simulink library "lib_FDM"  (R2019b)
settings: Solver=VariableStepAuto  StartTime=0.0  StopTime=10.0  RelTol=1e-3
values from neighbouring files (symbols this model uses):
  d = config.d_m    [computeTF.m]
undefined symbols (not defined in the file or in its folder): c_b_WGS, c_flat, c_grav, c_rot, c_rsma, Cd0, Cdcl, Cdcl2, Cl0, Cla, Cld, Cma, Cmd, Cmq, Cnb, Cnd, Cnr, Cra, Crd, Crp, Cy0, Cyb, Cyd, dmdt, Earth, HIL_Data, InitThrust, launchPos, me, mf, mp, Sref, tb, TF, theta0, WGS84
libraries: simulink_extras x14, $bdroot x7, simulink x5, lib_Fin_Deflections x3, aerolibasang x2, sharedtransform x1, aerolibtransform2 x1, aerolibbdyn x1, aerolibatmos2 x1, aerolibutil x1, aerolib6dof2 x1
(part 2 of 8)

== system lib_FDM/FDM/FDM_Linear/State_Integration ==
  FDM_States_Dot : Inport  OutDataTypeStr=Bus: FDM_States_Dot_Bus
  Simulation_Control : Inport  Port=2  OutDataTypeStr=Bus: Simulation_Ctrl_Bus
  States_Init : Inport  Port=3  OutDataTypeStr=Bus: States_Bus
  ATT_Integration : Subsystem
  Bus Creator : BusCreator  Inputs=4  OutDataTypeStr=Bus: FDM_States_Bus
  Bus Creator1 : BusCreator  Inputs=3  OutDataTypeStr=Bus: ATT_Euler_Bus
  Bus Creator2 : BusCreator  Inputs=3  OutDataTypeStr=Bus: Translation_States_Bus
  Bus Creator3 : BusCreator  Inputs=2  OutDataTypeStr=Bus: Airframe_States_Bus
  Bus Creator4 : BusCreator  Inputs=3  OutDataTypeStr=Bus: POS_WGS84_Bus
  Bus Creator5 : BusCreator  Inputs=3  OutDataTypeStr=Bus: POS_NED_Bus
  Bus Creator6 : BusCreator  Inputs=2  OutDataTypeStr=Bus: Position_States_Bus
  Bus Selector : BusSelector  OutputSignals=ATT_Euler_Dot.ATT_Dot_Phi_radDs,ATT_Euler_Dot.ATT_Dot_Theta_radDs,ATT_Euler_Dot.ATT_Dot_Psi_radDs
  Bus Selector1 : BusSelector  OutputSignals=Translation_States_Dot.ACC_x_B_mDs2,Translation_States_Dot.ACC_y_B_mDs2,Translation_States_Dot.ACC_z_B_mDs2
  Bus Selector2 : BusSelector  OutputSignals=Airframe_States_Dot.Motor_state_dot_percDs
  Bus Selector3 : BusSelector  OutputSignals=Position_States_Dot.POS_WGS84_Dot.POS_lambda_Dot_WGS84_radDs,Position_States_Dot.POS_WGS84_Dot.POS_mue_Dot_WGS84_radDs,Position_States_Dot.POS_WGS84_Dot.POS_h_Dot_WGS84_mDs
  Bus Selector4 : BusSelector  OutputSignals=Position_States_Dot.POS_NED_Dot.POS_x_Dot_NED_mDs,Position_States_Dot.POS_NED_Dot.POS_y_Dot_NED_mDs,Position_States_Dot.POS_NED_Dot.POS_z_Dot_NED_mDs
  Mass_Balance : Subsystem
  Motor_State_Integration : Subsystem
  POS_NED_Integrator : Subsystem
  POS_WGS84_Integrator : Subsystem
  Terminator1 : Terminator
  Terminator2 : Terminator
  Terminator3 : Terminator
  VEL_Integrator : Subsystem
  "FDM_States " : Outport  OutDataTypeStr=Bus: FDM_States_Bus  VectorParamsAs1DForOutWhenUnconnected=off
  wires:
  Mass_Balance/4(I_z_kgm2) -> Terminator3/1
  Mass_Balance/2(I_x_kgm2) -> Terminator1/1
  Mass_Balance/3(I_y_kgm2) -> Terminator2/1
  FDM_States_Dot/1 -> Bus Selector2/1, Bus Selector4/1, Bus Selector3/1, Bus Selector1/1, Bus Selector/1
  Bus Selector/1 -> ATT_Integration/3(phi_dot_radDs)  "<ATT_Dot_Phi_radDs>"
  Bus Selector/2 -> ATT_Integration/4(theta_dot_radDs)  "<ATT_Dot_Theta_radDs>"
  Bus Selector/3 -> ATT_Integration/5(psi_dot_radDs)  "<ATT_Dot_Psi_radDs>"
  Bus Creator/1 -> "FDM_States "/1
  ATT_Integration/3(psi_rad) -> Bus Creator1/3  "ATT_Psi_rad"
  ATT_Integration/2(theta_rad) -> Bus Creator1/2  "ATT_Theta_rad"
  ATT_Integration/1(phi_rad) -> Bus Creator1/1  "ATT_Phi_rad"
  Bus Creator1/1 -> Bus Creator/1  "Attitude_States"
  Simulation_Control/1 -> Motor_State_Integration/1(Simulation_Control), POS_NED_Integrator/1(Simulation_Control), POS_WGS84_Integrator/1(Simulation_Control), VEL_Integrator/1(Simulation_Control), ATT_Integration/1(Simulation_Control)
  States_Init/1 -> Motor_State_Integration/2(Initial_States), POS_NED_Integrator/2(Initial_States), POS_WGS84_Integrator/2(Initial_States), VEL_Integrator/2(Initial_States), ATT_Integration/2(Initial_States)
  Bus Creator2/1 -> Bus Creator/2  "Translation_States"
  VEL_Integrator/1(u_mDs) -> Bus Creator2/1  "VEL_u_K_R_E_B_mDs"
  VEL_Integrator/2(v_mDs) -> Bus Creator2/2  "VEL_v_K_R_E_B_mDs"
  VEL_Integrator/3(w_mDs) -> Bus Creator2/3  "VEL_w_K_R_E_B_mDs"
  Bus Selector1/3 -> VEL_Integrator/5(az_mDs2)  "<ACC_z_B_mDs2>"
  Bus Selector1/2 -> VEL_Integrator/4(ay_mDs2)  "<ACC_y_B_mDs2>"
  Bus Selector1/1 -> VEL_Integrator/3(ax_mDs2)  "<ACC_x_B_mDs2>"
  Bus Selector2/1 -> Motor_State_Integration/3(motor_state_dot_percDs)  "<Motor_state_dot_percDs>"
  Bus Creator3/1 -> Bus Creator/4  "Airframe_States"
  Motor_State_Integration/1(motor_state_perc) -> Mass_Balance/1(motor_state_perc), Bus Creator3/1  "motor_state_perc"
  Mass_Balance/1(mass_kg) -> Bus Creator3/2  "mass_kg"
  Bus Creator6/1 -> Bus Creator/3  "Position_States"
  Bus Creator4/1 -> Bus Creator6/1  "POS_WGS84"
  Bus Creator5/1 -> Bus Creator6/2  "POS_NED"
  POS_WGS84_Integrator/1(lambda_rad) -> Bus Creator4/1  "POS_lambda_ WGS84_rad"
  POS_WGS84_Integrator/2(mue_rad) -> Bus Creator4/2  "POS_mue_ WGS84_rad"
  POS_WGS84_Integrator/3(h_m) -> Bus Creator4/3  "POS_h_ WGS84_m"
  POS_NED_Integrator/1(x_m) -> Bus Creator5/1  "POS_x_NED_m"
  POS_NED_Integrator/2(y_m) -> Bus Creator5/2  "POS_y_NED_m"
  POS_NED_Integrator/3(z_m) -> Bus Creator5/3  "POS_z_NED_m"
  Bus Selector3/1 -> POS_WGS84_Integrator/3(lambda_dot_radDs)  "<POS_lambda_Dot_WGS84_radDs>"
  Bus Selector3/2 -> POS_WGS84_Integrator/4(mue_dot_radDs)  "<POS_mue_Dot_WGS84_radDs>"
  Bus Selector3/3 -> POS_WGS84_Integrator/5(h_dot_mDs)  "<POS_h_Dot_WGS84_mDs>"
  Bus Selector4/1 -> POS_NED_Integrator/3(x_dot_mDs)  "<POS_x_Dot_NED_mDs>"
  Bus Selector4/2 -> POS_NED_Integrator/4(y_dot_mDs)  "<POS_y_Dot_NED_mDs>"
  Bus Selector4/3 -> POS_NED_Integrator/5(z_dot_mDs)  "<POS_z_Dot_NED_mDs>"

== system lib_FDM/FDM/FDM_Sophisticated/Subsystem ==
  Servo Deflections : Inport  OutDataTypeStr=Bus: Control_Surface_Deflections_Bus
  Bus Selector : BusSelector  OutputSignals=Fin_1_Pos_rad,Fin_2_Pos_rad,Fin_3_Pos_rad,Fin_4_Pos_rad
  Constant1 : Constant  Value=HIL_Data.FDM.soph.bus1.unc_fin_def_roll
  Constant2 : Constant  Value=HIL_Data.FDM.soph.bus1.unc_fin_def_pitch
  Constant3 : Constant  Value=HIL_Data.FDM.soph.bus1.unc_fin_def_yaw
  Degrees to Radians : simulink_extras/Transformations/Degrees to Radians
  Degrees to Radians1 : simulink_extras/Transformations/Degrees to Radians
  Degrees to Radians2 : simulink_extras/Transformations/Degrees to Radians
  Sum : Sum  Inputs=|++
  Vector Concatenate : Concatenate  NumInputs=4
  Vector Concatenate1 : Concatenate  NumInputs=3
  control_allocation : Subsystem
  siB_cmd : Outport
  wires:
  Bus Selector/3 -> Vector Concatenate/3  "<Fin_3_Pos_rad>"
  Vector Concatenate/1 -> Sum/1
  Sum/1 -> siB_cmd/1  "siB_cmd"
  Bus Selector/4 -> Vector Concatenate/4  "<Fin_4_Pos_rad>"
  Bus Selector/1 -> Vector Concatenate/1  "<Fin_1_Pos_rad>"
  Servo Deflections/1 -> Bus Selector/1
  Bus Selector/2 -> Vector Concatenate/2  "<Fin_2_Pos_rad>"
  Constant2/1 -> Degrees to Radians1/1  "et_cmd"
  Constant3/1 -> Degrees to Radians2/1  "ze_cmd"
  Degrees to Radians/1 -> Vector Concatenate1/1
  control_allocation/1(siB_cmd) -> Sum/2
  Degrees to Radians1/1 -> Vector Concatenate1/2
  Constant1/1 -> Degrees to Radians/1  "xi_cmd"
  Vector Concatenate1/1 -> control_allocation/1(fin_cmd)  "fin_cmd"
  Degrees to Radians2/1 -> Vector Concatenate1/3

== system lib_FDM/FDM/FDM_Sophisticated/aerodynamics ==
  str_flow : Inport
  fin : Inport  Port=2
  wab : Inport  Port=3
  env_glbl : Inport  Port=4
  Bus Selector : BusSelector  OutputSignals=qdynB,MaB,alB,beB,hBE,wBIB_star
  Bus Selector1 : BusSelector  OutputSignals=afinB
  Bus Selector2 : BusSelector  OutputSignals=pBSB
  aerodynamic_via_lookup : Subsystem
  logic_base_drag : Subsystem
  aero : Outport  VectorParamsAs1DForOutWhenUnconnected=off
  wires:
  logic_base_drag/1(flag_base_drag) -> aerodynamic_via_lookup/9(flag_I_prp)
  env_glbl/1 -> logic_base_drag/1(env_glbl)
  aerodynamic_via_lookup/1(aero_bus) -> aero/1
  Bus Selector/6 -> aerodynamic_via_lookup/7(wBIB_star)  "<wBIB_star>"
  Bus Selector1/1 -> aerodynamic_via_lookup/8(afinB)  "<afinB>"
  Bus Selector/5 -> aerodynamic_via_lookup/6(hBE)  "<hBE>"
  Bus Selector/4 -> aerodynamic_via_lookup/5(beB)  "<beB>"
  Bus Selector/3 -> aerodynamic_via_lookup/4(alB)  "<alB>"
  Bus Selector/2 -> aerodynamic_via_lookup/3(MaB)  "<MaB>"
  Bus Selector/1 -> aerodynamic_via_lookup/2(qdynB)  "<qdynB>"
  Bus Selector2/1 -> aerodynamic_via_lookup/1(pBSB)  "<pBSB>"
  fin/1 -> Bus Selector1/1
  wab/1 -> Bus Selector2/1
  str_flow/1 -> Bus Selector/1

== system lib_FDM/FDM/FDM_Sophisticated/environment ==
  flight_dyn : Inport
  env_glbl : Inport  Port=2
  Bus Creator1 : BusCreator  Inputs=2
  Bus Creator2 : BusCreator  Inputs=2
  Bus Selector : BusSelector  OutputSignals=lon,lat,hBE
  Bus Selector1 : BusSelector  OutputSignals=atm_dyn_bus
  Saturation : Saturate  UpperLimit=inf  LowerLimit=eps
      settings: AttributesFormatString=|
      | %<UpperLimit>
      | %<LowerLimit>
  WGS84_Gravitation : Subsystem  mask{flg_omega_enabled=on}
      mask prompts: flg_omega_enabled "Zentripetalbeschleunigung mitberechnen"
      mask help:
      | Dieser Block berechnet die Gravitation für das idealisierte WGS84
      | Ellipsoid. Die Berechnung ist hierbei nach dem Technical Report
      | "Department of Defense World Geodetic System 1984", NIMA TR8350.2,
      | Third Edition, Amendment 1 vom 3 Januar 2000 implementiert.
      | Das Modell ist gültig für alle Höhen über dem WGS84 Referenzellipsoid, und
      | ist somit der reinen Taylorexpansion des Somigliana Modells überlegen
      | (siehe Kapitel 4.3 des WGS84 reports).
      |
      | ---------------------------------------------------------------------------
      | Longitude [rad]: Nach WGS84 definierte Geodätische Länge.  (lambda)
      | Lattitude [rad]: Nach WGS84 definierte Geodätische Breite. (phi)
      | Height [m]: Höhe über dem WGS84 Referenzellipsoid.
      mask init:
      | [ c_rsma, c_b_WGS, c_grav, c_rot] = init_WGS84_Gravitationsmodell();
  atmosphere_static_ISO_2533 : Subsystem
  convert_to_local_frame : Subsystem
  env : Outport  VectorParamsAs1DForOutWhenUnconnected=off
  wires:
  Bus Selector1/1 -> Bus Creator1/2  "<atm_dyn_bus>"
  env_glbl/1 -> atmosphere_static_ISO_2533/2(env_glbl), Bus Selector1/1
  atmosphere_static_ISO_2533/1(atm_stat) -> Bus Creator1/1  "atm_stat_bus"
  Saturation/1 -> WGS84_Gravitation/3(h)
  Bus Creator1/1 -> Bus Creator2/2  "atm_bus"
  Bus Selector/2 -> WGS84_Gravitation/2(lat)  "<lat>"
  Bus Creator2/1 -> env/1  "env_bus"
  Bus Selector/3 -> Saturation/1, atmosphere_static_ISO_2533/1(hBE)  "<hBE>"
  Bus Selector/1 -> WGS84_Gravitation/1(lon)  "<lon>"
  WGS84_Gravitation/1(gE) -> convert_to_local_frame/1(gE)
  flight_dyn/1 -> Bus Selector/1
  convert_to_local_frame/1(gBG) -> Bus Creator2/1

== system lib_FDM/FDM/FDM_Sophisticated/fin_actuators ==
  cmd : Inport
  Bus Creator3 : BusCreator  Inputs=7
  Bus Selector : BusSelector  OutputSignals=siB_cmd
  Constant7 : Constant  Value=HIL_Data.FDM.soph.bus1.tRRR
  Demux : Demux
  Rudder : Subsystem  mask{siB_max=HIL_Data.FDM.soph.bus1.siB_max, siB_min=HIL_Data.FDM.soph.bus1.siB_min, d_siB_max=HIL_Data.FDM.soph.bus1.d_siB_max, d_siB_min=HIL_Data.FDM.soph.bus1.d_siB_min, dd_siB_max=HIL_Data.FDM.soph.bus1.dd_siB_max, dd_siB_min=HIL_Data.FDM.soph.bus1.dd_siB_min, omega=HIL_Data.FDM.soph.bus1.act_omega, dmp=HIL_Data.FDM.soph.bus1.act_dmp, unc_bl=HIL_Data.FDM.soph.bus1.unc_act_bl, unc_scale=HIL_Data.FDM.soph.bus1.unc_act_scale, unc_off=HIL_Data.FDM.soph.bus1.unc_act_off, siB_0=HIL_Data.FDM.soph.bus1.siB_0, d_siB_0=HIL_Data.FDM.soph.bus1.d_siB_0}
      mask prompts: siB_max "Obere Limitierung des Ruderstellwinkels in [rad]"; siB_min "Untere Limitierung des Ruderstellwinkels in [rad]"; d_siB_max "Obere Limitierung der Ruderstellwinkelgeschwindigkeit in [rad/s]"; d_siB_min "Untere Limitierung der Ruderstellwinkelgeschwindigkeit in [rad/s]"; dd_siB_max "Obere Limitierung der Ruderstellwinkelbeschleunigung in [rad/s^2]"; dd_siB_min "Untere Limitierung der Ruderstellwinkelbeschleunigung in [rad/s^2]"; omega "Eckfrequenz in [Hz]"; dmp "Dämpfung in [kg/s]"; unc_bl "Rückschlag des Aktuators (Backlash) in [rad]"; unc_scale "Skalenfehler in [-]"; unc_off "Versatz (Offset) in [rad]"; siB_0 "Startwert Ruderwinkel in [rad]"; d_siB_0 "Startwert Ruderwinkelgeschwindigkeiten in [rad/s]"
      mask DialogControl ParameterGroupVar Prompt: Limitierungen
      mask DialogControl Container3 Prompt: Dynamik
      mask DialogControl Container4 Prompt: Aktuatorfehler
      mask DialogControl Container5 Prompt: Startwerte
  Rudder1 : Subsystem  mask{siB_max=HIL_Data.FDM.soph.bus1.siB_max, siB_min=HIL_Data.FDM.soph.bus1.siB_min, d_siB_max=HIL_Data.FDM.soph.bus1.d_siB_max, d_siB_min=HIL_Data.FDM.soph.bus1.d_siB_min, dd_siB_max=HIL_Data.FDM.soph.bus1.dd_siB_max, dd_siB_min=HIL_Data.FDM.soph.bus1.dd_siB_min, omega=HIL_Data.FDM.soph.bus1.act_omega, dmp=HIL_Data.FDM.soph.bus1.act_dmp, unc_bl=HIL_Data.FDM.soph.bus1.unc_act_bl, unc_scale=HIL_Data.FDM.soph.bus1.unc_act_scale, unc_off=HIL_Data.FDM.soph.bus1.unc_act_off, siB_0=HIL_Data.FDM.soph.bus1.siB_0, d_siB_0=HIL_Data.FDM.soph.bus1.d_siB_0}
      mask prompts: siB_max "Obere Limitierung des Ruderstellwinkels in [rad]"; siB_min "Untere Limitierung des Ruderstellwinkels in [rad]"; d_siB_max "Obere Limitierung der Ruderstellwinkelgeschwindigkeit in [rad/s]"; d_siB_min "Untere Limitierung der Ruderstellwinkelgeschwindigkeit in [rad/s]"; dd_siB_max "Obere Limitierung der Ruderstellwinkelbeschleunigung in [rad/s^2]"; dd_siB_min "Untere Limitierung der Ruderstellwinkelbeschleunigung in [rad/s^2]"; omega "Eckfrequenz in [Hz]"; dmp "Dämpfung in [kg/s]"; unc_bl "Rückschlag des Aktuators (Backlash) in [rad]"; unc_scale "Skalenfehler in [-]"; unc_off "Versatz (Offset) in [rad]"; siB_0 "Startwert Ruderwinkel in [rad]"; d_siB_0 "Startwert Ruderwinkelgeschwindigkeiten in [rad/s]"
      mask DialogControl ParameterGroupVar Prompt: Limitierungen
      mask DialogControl Container3 Prompt: Dynamik
      mask DialogControl Container4 Prompt: Aktuatorfehler
      mask DialogControl Container5 Prompt: Startwerte
  Rudder2 : Subsystem  mask{siB_max=HIL_Data.FDM.soph.bus1.siB_max, siB_min=HIL_Data.FDM.soph.bus1.siB_min, d_siB_max=HIL_Data.FDM.soph.bus1.d_siB_max, d_siB_min=HIL_Data.FDM.soph.bus1.d_siB_min, dd_siB_max=HIL_Data.FDM.soph.bus1.dd_siB_max, dd_siB_min=HIL_Data.FDM.soph.bus1.dd_siB_min, omega=HIL_Data.FDM.soph.bus1.act_omega, dmp=HIL_Data.FDM.soph.bus1.act_dmp, unc_bl=HIL_Data.FDM.soph.bus1.unc_act_bl, unc_scale=HIL_Data.FDM.soph.bus1.unc_act_scale, unc_off=HIL_Data.FDM.soph.bus1.unc_act_off, siB_0=HIL_Data.FDM.soph.bus1.siB_0, d_siB_0=HIL_Data.FDM.soph.bus1.d_siB_0}
      mask prompts: siB_max "Obere Limitierung des Ruderstellwinkels in [rad]"; siB_min "Untere Limitierung des Ruderstellwinkels in [rad]"; d_siB_max "Obere Limitierung der Ruderstellwinkelgeschwindigkeit in [rad/s]"; d_siB_min "Untere Limitierung der Ruderstellwinkelgeschwindigkeit in [rad/s]"; dd_siB_max "Obere Limitierung der Ruderstellwinkelbeschleunigung in [rad/s^2]"; dd_siB_min "Untere Limitierung der Ruderstellwinkelbeschleunigung in [rad/s^2]"; omega "Eckfrequenz in [Hz]"; dmp "Dämpfung in [kg/s]"; unc_bl "Rückschlag des Aktuators (Backlash) in [rad]"; unc_scale "Skalenfehler in [-]"; unc_off "Versatz (Offset) in [rad]"; siB_0 "Startwert Ruderwinkel in [rad]"; d_siB_0 "Startwert Ruderwinkelgeschwindigkeiten in [rad/s]"
      mask DialogControl ParameterGroupVar Prompt: Limitierungen
      mask DialogControl Container3 Prompt: Dynamik
      mask DialogControl Container4 Prompt: Aktuatorfehler
      mask DialogControl Container5 Prompt: Startwerte
  Rudder3 : Subsystem  mask{siB_max=HIL_Data.FDM.soph.bus1.siB_max, siB_min=HIL_Data.FDM.soph.bus1.siB_min, d_siB_max=HIL_Data.FDM.soph.bus1.d_siB_max, d_siB_min=HIL_Data.FDM.soph.bus1.d_siB_min, dd_siB_max=HIL_Data.FDM.soph.bus1.dd_siB_max, dd_siB_min=HIL_Data.FDM.soph.bus1.dd_siB_min, omega=HIL_Data.FDM.soph.bus1.act_omega, dmp=HIL_Data.FDM.soph.bus1.act_dmp, unc_bl=HIL_Data.FDM.soph.bus1.unc_act_bl, unc_scale=HIL_Data.FDM.soph.bus1.unc_act_scale, unc_off=HIL_Data.FDM.soph.bus1.unc_act_off, siB_0=HIL_Data.FDM.soph.bus1.siB_0, d_siB_0=HIL_Data.FDM.soph.bus1.d_siB_0}
      mask prompts: siB_max "Obere Limitierung des Ruderstellwinkels in [rad]"; siB_min "Untere Limitierung des Ruderstellwinkels in [rad]"; d_siB_max "Obere Limitierung der Ruderstellwinkelgeschwindigkeit in [rad/s]"; d_siB_min "Untere Limitierung der Ruderstellwinkelgeschwindigkeit in [rad/s]"; dd_siB_max "Obere Limitierung der Ruderstellwinkelbeschleunigung in [rad/s^2]"; dd_siB_min "Untere Limitierung der Ruderstellwinkelbeschleunigung in [rad/s^2]"; omega "Eckfrequenz in [Hz]"; dmp "Dämpfung in [kg/s]"; unc_bl "Rückschlag des Aktuators (Backlash) in [rad]"; unc_scale "Skalenfehler in [-]"; unc_off "Versatz (Offset) in [rad]"; siB_0 "Startwert Ruderwinkel in [rad]"; d_siB_0 "Startwert Ruderwinkelgeschwindigkeiten in [rad/s]"
      mask DialogControl ParameterGroupVar Prompt: Limitierungen
      mask DialogControl Container3 Prompt: Dynamik
      mask DialogControl Container4 Prompt: Aktuatorfehler
      mask DialogControl Container5 Prompt: Startwerte
  Vector Concatenate1 : Concatenate  NumInputs=4
  Vector Concatenate2 : Concatenate  NumInputs=4
  Vector Concatenate3 : Concatenate  NumInputs=4
  control_allocation : Subsystem
  fin : Outport  VectorParamsAs1DForOutWhenUnconnected=off
  wires:
  control_allocation/4(dd_finB) -> Bus Creator3/5
  control_allocation/3(d_finB) -> Bus Creator3/4
  control_allocation/2(finB) -> Bus Creator3/3
  control_allocation/1(Tr3r4) -> Bus Creator3/2
  Vector Concatenate3/1 -> control_allocation/3(dd_siB), Bus Creator3/6  "dd_siB"
  Vector Concatenate2/1 -> control_allocation/2(d_siB), Bus Creator3/7  "d_siB"
  Vector Concatenate1/1 -> control_allocation/1(siB), Bus Creator3/1  "siB"
  Bus Creator3/1 -> fin/1  "fin_bus"
  Rudder/1(siB) -> Vector Concatenate1/1
  Rudder/3(dd_siB) -> [dd_siB1]
  Demux/2 -> Rudder1/1(siB_c)
  Rudder2/3(dd_siB) -> [dd_siB3]
  Rudder/2(d_siB) -> [d_siB1]
  Rudder3/3(dd_siB) -> [dd_siB4]
  Rudder1/3(dd_siB) -> [dd_siB2]
  Rudder1/1(siB) -> Vector Concatenate1/2
  [dd_siB1] -> Vector Concatenate3/1
  cmd/1 -> Bus Selector/1
  [dd_siB3] -> Vector Concatenate3/3
  [dd_siB4] -> Vector Concatenate3/4
  Demux/1 -> Rudder/1(siB_c)
  Rudder3/2(d_siB) -> [d_siB4]
  Demux/3 -> Rudder2/1(siB_c)
  [dd_siB2] -> Vector Concatenate3/2
  Constant7/1 -> Rudder/2(tRRR), Rudder2/2(tRRR), Rudder3/2(tRRR), Rudder1/2(tRRR)
  [d_siB2] -> Vector Concatenate2/2
  Bus Selector/1 -> Demux/1  "<siB_cmd>"
  [d_siB1] -> Vector Concatenate2/1
  [d_siB4] -> Vector Concatenate2/4
  Rudder2/1(siB) -> Vector Concatenate1/3
  Rudder1/2(d_siB) -> [d_siB2]
  Rudder3/1(siB) -> Vector Concatenate1/4
  Rudder2/2(d_siB) -> [d_siB3]
  Demux/4 -> Rudder3/1(siB_c)
  [d_siB3] -> Vector Concatenate2/3

== system lib_FDM/FDM/FDM_Sophisticated/forces_moments ==
  aero : Inport
  motion_kin : Inport  Port=2
  grav : Inport  Port=3
  prp : Inport  Port=4
  External_FM : Inport  Port=5
  Add : Sum  Inputs=++++
  Add1 : Sum  Inputs=+++
  Bus Creator : BusCreator  Inputs=2
  Bus Selector : BusSelector  OutputSignals=FBAB,MBAB
  Bus Selector1 : BusSelector  OutputSignals=TGB
  Bus Selector2 : BusSelector  OutputSignals=FBGG
  Bus Selector3 : BusSelector  OutputSignals=FBPB,MBPB
  Bus Selector5 : BusSelector  OutputSignals=Disturbance_Force_N,Disturbance_Moment_Nm
  Math Function : Math  Operator=transpose  SaturateOnIntegerOverflow=on
  Product : Product  Multiplication=Matrix(*)
  for_mom_bus : Outport  VectorParamsAs1DForOutWhenUnconnected=off
  wires:
  Bus Selector3/2 -> Add1/2  "<MBPB>"
  Bus Creator/1 -> for_mom_bus/1  "for_mom_bus"
  Bus Selector3/1 -> Add/3  "<FBPB>"
  Bus Selector/2 -> Add1/1  "<MBAB>"
  Add1/1 -> Bus Creator/2  "MBTB"
  grav/1 -> Bus Selector2/1
  Add/1 -> Bus Creator/1  "FBTB"
  motion_kin/1 -> Bus Selector1/1
  prp/1 -> Bus Selector3/1
  Product/1 -> Add/2  "FBGB"
  aero/1 -> Bus Selector/1
  Math Function/1 -> Product/1  "TBG"
  Bus Selector1/1 -> Math Function/1  "<TGB>"
  Bus Selector2/1 -> Product/2  "<FBGG>"
  Bus Selector/1 -> Add/1  "<FBAB>"
  External_FM/1 -> Bus Selector5/1
  Bus Selector5/1 -> Add/4  "<Disturbance_Force_N>"
  Bus Selector5/2 -> Add1/3  "<Disturbance_Moment_Nm>"

== system lib_FDM/FDM/FDM_Sophisticated/gravity ==
  env : Inport
  wab : Inport  Port=2
  Bus Creator3 : BusCreator  Inputs=1
  Bus Selector : BusSelector  OutputSignals=gBG,atm_bus.atm_stat_bus.hBE
  Bus Selector1 : BusSelector  OutputSignals=mB
  Product : Product
  launch_rail : Subsystem
  grav : Outport  VectorParamsAs1DForOutWhenUnconnected=off
  wires:
  env/1 -> Bus Selector/1
  Bus Selector1/1 -> Product/2  "<mB>"
  wab/1 -> Bus Selector1/1
  Bus Creator3/1 -> grav/1  "grav_bus"
  Product/1 -> Bus Creator3/1  "FBGG"
  Bus Selector/1 -> launch_rail/1(gBG_c)  "<gBG>"
  Bus Selector/2 -> launch_rail/2(hBE)  "<hBE>"
  launch_rail/1(gBG) -> Product/1

== system lib_FDM/FDM/FDM_Sophisticated/input ==
  siB_cmd : Inport
  Bus Creator2 : BusCreator  Inputs=1
  cmd_bus : Outport  VectorParamsAs1DForOutWhenUnconnected=off
  wires:
  Bus Creator2/1 -> cmd_bus/1  "cmd_bus"
  siB_cmd/1 -> Bus Creator2/1

== system lib_FDM/FDM/FDM_Sophisticated/motion_kinematics ==
  flight_dyn : Inport
  Bus Creator : BusCreator  Inputs=7
  Bus Selector : BusSelector  OutputSignals=lat,lon,qIB
  calc_motion_kinematics : Subsystem
  motion_kin : Outport  VectorParamsAs1DForOutWhenUnconnected=off
  wires:
  calc_motion_kinematics/7(TIB) -> Bus Creator/7
  calc_motion_kinematics/6(wEGG) -> Bus Creator/6
  calc_motion_kinematics/5(TEG) -> Bus Creator/5
  calc_motion_kinematics/4(TGB) -> Bus Creator/4
  calc_motion_kinematics/3(TEB) -> Bus Creator/3
  calc_motion_kinematics/2(TIE) -> Bus Creator/2
  calc_motion_kinematics/1(wIEE) -> Bus Creator/1
  Bus Selector/3 -> calc_motion_kinematics/3(qIB)  "<qIB>"
  Bus Selector/2 -> calc_motion_kinematics/2(lon)  "<lon>"
  Bus Selector/1 -> calc_motion_kinematics/1(lat)  "<lat>"
  Bus Creator/1 -> motion_kin/1  "motion_kin_bus"
  flight_dyn/1 -> Bus Selector/1

== system lib_FDM/FDM/FDM_Sophisticated/propulsion ==
  env_glbl : Inport
  wab : Inport  Port=2
  Bus Creator1 : BusCreator  Inputs=3
  prp_look_up : Subsystem
  prp_uncertainty : Subsystem
  prp : Outport  VectorParamsAs1DForOutWhenUnconnected=off
  wires:
  prp_look_up/1(dmB) -> Bus Creator1/1
  wab/1 -> prp_uncertainty/2(wab)
  prp_uncertainty/1(FBPB) -> Bus Creator1/2
  prp_uncertainty/2(MBPB) -> Bus Creator1/3
  env_glbl/1 -> prp_look_up/1(env_glbl_bus)
  prp_look_up/2(FBPM) -> prp_uncertainty/1(FBPM)
  Bus Creator1/1 -> prp/1  "prp_bus"

== system lib_FDM/FDM/FDM_Sophisticated/quaternion_to_euler_angles ==
  note: Um numerische Probleme zu
      | vermeiden, wird hier eine Saturiierung
      | benutzt.
  note: Outputs [size]:
      |
      | roll angle [1]
      | pitch angle [1]
      | yaw angle [1]
  note: Inputs [size]:
      |
      | quaternion [4]
  q : Inport  PortDimensions=4
  Add : Sum
  Add1 : Sum  Inputs=+--
  Add2 : Sum  Inputs=+-
  Add3 : Sum
  Add4 : Sum  Inputs=+--
  Complex to Real-Imag : ComplexToRealImag  Output=Real
  Constant : Constant  Value=0.5
  Constant1 : Constant  Value=0.5
  Demux : Demux
  Gain : Gain  Gain=2
  Product{,1..9} (10 alike) : Product
  Saturation : Saturate  UpperLimit=1  LowerLimit=-1
      settings: AttributesFormatString=|
      | %<UpperLimit>
      | %<LowerLimit>
  Trigonometric Function : Trigonometry  Operator=atan2
  Trigonometric Function1 : Trigonometry  Operator=asin
  Trigonometric Function2 : Trigonometry  Operator=atan2
  Vector Concatenate : Concatenate  NumInputs=3
  eulx : Outport  VectorParamsAs1DForOutWhenUnconnected=off
  wires:
  Vector Concatenate/1 -> Complex to Real-Imag/1
  Complex to Real-Imag/1 -> eulx/1
  Trigonometric Function2/1 -> Vector Concatenate/3
  Trigonometric Function1/1 -> Vector Concatenate/2
  Trigonometric Function/1 -> Vector Concatenate/1
  Add/1 -> Trigonometric Function/1
  Product1/1 -> Add/2
  Product/1 -> Add/1
  Product3/1 -> Add1/3
  Product2/1 -> Add1/2
  Product5/1 -> Add2/2
  Product4/1 -> Add2/1
  Product7/1 -> Add3/2
  Product6/1 -> Add3/1
  Add3/1 -> Trigonometric Function2/1
  Add4/1 -> Trigonometric Function2/2
  Add2/1 -> Gain/1
  Add1/1 -> Trigonometric Function/2
  q/1 -> Demux/1
  Demux/4 -> Product7/2, Product4/2, Product/2  "4"
  Demux/1 -> Product2/2, Product2/1, Product/1, Product6/1, Product5/1  "1"
  Demux/2 -> Product4/1, Product3/2, Product3/1, Product1/1, Product8/2, Product8/1, Product6/2  "2"
  Constant/1 -> Add1/1
  Product9/1 -> Add4/3
  Product8/1 -> Add4/2
  Constant1/1 -> Add4/1
  Demux/3 -> Product9/2, Product9/1, Product7/1, Product1/2, Product5/2  "3"
  Gain/1 -> Saturation/1
  Saturation/1 -> Trigonometric Function1/1

== system lib_FDM/FDM/FDM_Sophisticated/rb_eom ==
  mot_kin : Inport
  for_mom : Inport  Port=2
  wab : Inport  Port=3
  Bus Creator : BusCreator  Inputs=12
  calc_bus_flight_dyn_bus_entries : Subsystem
  eom_6dof : Subsystem
  flight_dyn : Outport  VectorParamsAs1DForOutWhenUnconnected=off
  wires:
  calc_bus_flight_dyn_bus_entries/12(vBIB) -> Bus Creator/12
  calc_bus_flight_dyn_bus_entries/11(euIB) -> Bus Creator/11
  calc_bus_flight_dyn_bus_entries/10(pBII) -> Bus Creator/10
  eom_6dof/1(eom) -> calc_bus_flight_dyn_bus_entries/2(eom)
  wab/1 -> eom_6dof/2(wab)
  for_mom/1 -> eom_6dof/1(for_mom)
  Bus Creator/1 -> flight_dyn/1  "flight_dyn_bus"
  calc_bus_flight_dyn_bus_entries/9(d_vBII) -> Bus Creator/9
  calc_bus_flight_dyn_bus_entries/8(d_wBIB) -> Bus Creator/8
  calc_bus_flight_dyn_bus_entries/7(wBIB) -> Bus Creator/7
  calc_bus_flight_dyn_bus_entries/6(qIB) -> Bus Creator/6
  calc_bus_flight_dyn_bus_entries/5(vBII) -> Bus Creator/5
  calc_bus_flight_dyn_bus_entries/4(hBE) -> Bus Creator/4
  calc_bus_flight_dyn_bus_entries/3(lat) -> Bus Creator/3
  calc_bus_flight_dyn_bus_entries/2(lon) -> Bus Creator/2
  calc_bus_flight_dyn_bus_entries/1(aBIB) -> Bus Creator/1
  mot_kin/1 -> calc_bus_flight_dyn_bus_entries/1(mot_kin)

== system lib_FDM/FDM/FDM_Sophisticated/stream_flow ==
  flight_dyn : Inport
  motion_kin : Inport  Port=2
  env : Inport  Port=3
  Bus Selector1 : BusSelector  OutputSignals=atm_bus.atm_stat_bus.rho,atm_bus.atm_stat_bus.sos,atm_bus.atm_stat_bus.hBE,atm_bus.atm_dyn_bus.vWEG
  Bus Selector2 : BusSelector  OutputSignals=vBII,pBII,wBIB
  Bus Selector3 : BusSelector  OutputSignals=TIB,wIEE,TIE,TGB
  calc_stream_flow : Subsystem
  str_flow : Outport  VectorParamsAs1DForOutWhenUnconnected=off
  wires:
  Bus Selector3/4 -> calc_stream_flow/4(TGB)  "<TGB>"
  Bus Selector1/4 -> calc_stream_flow/11(vWEG)  "<vWEG>"
  Bus Selector2/2 -> calc_stream_flow/6(pBII)  "<pBII>"
  calc_stream_flow/1(str_flow) -> str_flow/1
  Bus Selector1/3 -> calc_stream_flow/10(hBE)  "<hBE>"
  Bus Selector1/2 -> calc_stream_flow/9(sos)  "<sos>"
  Bus Selector1/1 -> calc_stream_flow/8(rho)  "<rho>"
  Bus Selector2/3 -> calc_stream_flow/7(wBIB)  "<wBIB>"
  Bus Selector2/1 -> calc_stream_flow/5(vBII)  "<vBII>"
  Bus Selector3/3 -> calc_stream_flow/3(TIE)  "<TIE>"
  Bus Selector3/2 -> calc_stream_flow/2(wIEE)  "<wIEE>"
  Bus Selector3/1 -> calc_stream_flow/1(TIB)  "<TIB>"
  env/1 -> Bus Selector1/1
  flight_dyn/1 -> Bus Selector2/1
  motion_kin/1 -> Bus Selector3/1

== system lib_FDM/FDM/FDM_Sophisticated/tmp ==
  Bus Creator1 : BusCreator  Inputs=5
  Time : Subsystem
  weather : Subsystem
  env_glbl_bus : Outport
  wires:
  Time/1(T_sim_glbl) -> Bus Creator1/1
  weather/3(e_pa) -> Bus Creator1/5
  weather/2(e_Tmp) -> Bus Creator1/4
  Time/2(T_sim_lnch) -> Bus Creator1/2
  Bus Creator1/1 -> env_glbl_bus/1  "env_glbl_bus"
  weather/1(atm_dyn) -> Bus Creator1/3

== system lib_FDM/FDM/FDM_Sophisticated/weight_and_balance ==
  prp : Inport
  env_glb : Inport  Port=2
  Bus Creator1 : BusCreator  Inputs=4
  Bus Selector2 : BusSelector  OutputSignals=T_sim_glbl,T_sim_lnch
  Subtract : Sum  Inputs=+-
  center_of_gravity : Subsystem
  d_moi : Subsystem
  mass : Subsystem
  mass_uncertainty : Subsystem
  moi : Subsystem
  wab : Outport  VectorParamsAs1DForOutWhenUnconnected=off
  wires:
  d_moi/1(d_JBBB) -> Bus Creator1/4
  prp/1 -> d_moi/1(prp)
  Subtract/1 -> mass/1(sim_time_launch)
  mass/1(mB_c) -> mass_uncertainty/1(mB_c)
  mass_uncertainty/1(mB) -> Bus Creator1/1, center_of_gravity/1(mB)
  mass/2(mM) -> center_of_gravity/2(mM), moi/2(mM)
  moi/1(JBBB) -> Bus Creator1/3
  center_of_gravity/1(pBSB) -> Bus Creator1/2, moi/1(pBPB)
  Bus Creator1/1 -> wab/1  "wab_bus"
  env_glb/1 -> Bus Selector2/1
  Bus Selector2/1 -> Subtract/1  "<T_sim_glbl>"
  Bus Selector2/2 -> Subtract/2  "<T_sim_lnch>"

== system lib_FDM/FDM/FDM_Student/Aerodynamics ==
  "delta Y " : Inport
  delta P : Inport  Port=2
  delta R : Inport  Port=3
  - : Subsystem
  DCM_Body_To_Wind : MATLAB Function  TreatAsAtomicUnit=on
  DCM_Wind_To_Body : MATLAB Function  TreatAsAtomicUnit=on
  DCM_Wind_To_Body1 : MATLAB Function  TreatAsAtomicUnit=on
  Force Calc : Subsystem
  Gravity : Subsystem
  Moment Calc : Subsystem
  Mux : Mux  Inputs=3
      settings: DisplayOption=signals
  Mux1 : Mux  Inputs=3
      settings: DisplayOption=signals
  Sum1 : Sum  Inputs=|+++
  To Workspace : ToWorkspace  VariableName=Mb  SaveFormat=Structure  SampleTime=-1
  To Workspace1 : ToWorkspace  VariableName=Fb  SaveFormat=Structure  SampleTime=-1
  "[Fxb Fyb Fzb]" : Outport  VectorParamsAs1DForOutWhenUnconnected=off
  "[Mxb Myb Mzb]" : Outport  Port=2  VectorParamsAs1DForOutWhenUnconnected=off
  tag scope: GravityBodyAxis=global
  wires:
  Gravity/1(Gravity) -> Sum1/3, [GravityBodyAxis]
  delta R/1 -> Moment Calc/3(delta_R)
  [beta] -> Moment Calc/6(beta), Force Calc/1(beta)
  "delta Y "/1 -> Force Calc/2(delta Y), Moment Calc/7(delta Y)
  delta P/1 -> Moment Calc/5(delta P), Force Calc/4(delta P)
  [AOA] -> Force Calc/3(AOA), Moment Calc/4(alpha)
  Force Calc/1(D) -> Mux/1
  Force Calc/2(Y) -> Mux/2
  Force Calc/3(L) -> Mux/3
  Moment Calc/1(L) -> Mux1/1  "Mx"
  Moment Calc/2(M) -> Mux1/2  "My"
  Moment Calc/3(N) -> Mux1/3  "Mz"
  [AOA] -> DCM_Wind_To_Body/1(alpha)
  [beta] -> DCM_Wind_To_Body/2(beta)
  DCM_Wind_To_Body/1(MB) -> To Workspace/1, "[Mxb Myb Mzb]"/1
  Mux1/1 -> DCM_Wind_To_Body/3(MW)  "M_Wind"
  Mux/1 -> DCM_Wind_To_Body1/3(FW)  "F_Wind"
  [AOA] -> DCM_Wind_To_Body1/1(alpha)
  [beta] -> DCM_Wind_To_Body1/2(beta)
  [q] -> Force Calc/5(q), Moment Calc/8(q)
  [BodyVel] -> Moment Calc/2(Vb)
  Sum1/1 -> To Workspace1/1, "[Fxb Fyb Fzb]"/1  "Fb"
  -/1(Thrust) -> Sum1/1
  DCM_Wind_To_Body1/1(FB) -> Sum1/2
  [AOA] -> DCM_Body_To_Wind/1(alpha)
  [beta] -> DCM_Body_To_Wind/2(beta)
  [BodyAngularVel] -> DCM_Body_To_Wind/3(wb)
  DCM_Body_To_Wind/1(w_Wind) -> Moment Calc/1(w_wind)

== system lib_FDM/FDM/FDM_Student/Global Calculations ==
  note: Atmospheric calculations
  note: Aerodynamic parameters
  note: Mass and CG
  Abs : Abs
  CalcMass : MATLAB Function  TreatAsAtomicUnit=on
  "Calculate AOA, Sideslip and Airspeed" : Subsystem
  Clock : Clock
  Constant : Constant  Value=mf
  Constant1 : Constant  Value=mp
  Constant2 : Constant  Value=dmdt
  Constant3 : Constant  Value=me
  Constant4 : Constant  Value=tb
  Direction Cosine Matrix Body to Wind : aerolibtransform2/Direction Cosine Matrix Body to Wind
      settings: SourceProductName=Aerospace Blockset  SourceProductBaseCode=AE
  Dynamic Pressure : aerolibasang/Dynamic Pressure
  Estimate Center of Gravity : aerolibbdyn/Estimate Center of Gravity  fmass=mf  emass=me  fcg=xcgf  ecg=xcge
      settings: SourceProductName=Aerospace Blockset  SourceProductBaseCode=AE
  Gain : Gain
  ISA Atmosphere Model : aerolibatmos2/ISA Atmosphere Model  custom=off  g=9.80665  gamma=1.4  R=287.0531  L=0.0065  h_trop=11000  h_strat=20000  rho0=1.225  P0=101325  T0=288.15  h0=0
      settings: SourceProductName=Aerospace Blockset
  Invert 3x3 Matrix : aerolibutil/Invert  3x3 Matrix
  Mux : Mux  Inputs=2
  Selector : Selector  InputPortWidth=3  IndexOptions=Index vector (dialog)  Indices=[3]  OutputSizes=1
  Selector1 : Selector  InputPortWidth=3  IndexOptions=Index vector (dialog)  Indices=[1]  OutputSizes=1
  Terminator{1..3,9..11} (6 alike) : Terminator
  "To " : ToWorkspace  VariableName=alpha  SampleTime=-1
  To 1 : ToWorkspace  VariableName=beta  SampleTime=-1
  To Workspace2 : ToWorkspace  VariableName=mass  SampleTime=-1
  To Workspace3 : ToWorkspace  VariableName=x_cg  SaveFormat=Timeseries  SampleTime=-1
  To Workspace4 : ToWorkspace  VariableName=mass_dot  SampleTime=-1
  To Workspace5 : ToWorkspace  VariableName=qdyn  SampleTime=-1
  tag scope: AOA=global, BodyMass=global, Xcg=global, beta=global, dmdt=global, q=global
  wires:
  ISA Atmosphere Model/2 -> Terminator10/1
  ISA Atmosphere Model/1 -> Terminator1/1
  "Calculate AOA, Sideslip and Airspeed"/3(V) -> Terminator9/1
  "Calculate AOA, Sideslip and Airspeed"/2(beta) -> To 1/1, [beta], Mux/2
  ISA Atmosphere Model/3 -> Terminator11/1
  Selector/1 -> ISA Atmosphere Model/1
  ISA Atmosphere Model/4 -> Dynamic Pressure/2
  Dynamic Pressure/1 -> To Workspace5/1, [q]
  Mux/1 -> Direction Cosine Matrix Body to Wind/1
  [BodyVel] -> Abs/1, "Calculate AOA, Sideslip and Airspeed"/1(In1)
  Direction Cosine Matrix Body to Wind/1 -> Invert 3x3 Matrix/1
  "Calculate AOA, Sideslip and Airspeed"/1(AOA) -> "To "/1, [AOA], Mux/1
  [PosWGS] -> Gain/1
  Estimate Center of Gravity/2 -> Terminator2/1
  Estimate Center of Gravity/1 -> Selector1/1, [Xcg]
  CalcMass/1(m) -> Estimate Center of Gravity/1, To Workspace2/1, [BodyMass]
  CalcMass/2(m_dot) -> Estimate Center of Gravity/2, [dmdt], To Workspace4/1
  Clock/1 -> CalcMass/1(t)
  Selector1/1 -> To Workspace3/1
  Constant/1 -> CalcMass/2(mf)
  Constant1/1 -> CalcMass/3(mp)
  Constant3/1 -> CalcMass/4(me)
  Constant2/1 -> CalcMass/5(dmdt)
  Constant4/1 -> CalcMass/6(tb)
  Abs/1 -> Dynamic Pressure/1
  Invert 3x3 Matrix/1 -> Terminator3/1
  Gain/1 -> Selector/1

== system lib_FDM/FDM/FDM_Basic/Motion_Kinematics/Drag ==
  alpha : Inport
  beta : Inport  Port=2
  Enable : EnablePort
  Constant : Constant  Value=-1
  Constant1 : Constant  Value=-1
  Constant2 : Constant  Value=-1
  Terminator : Terminator
  Terminator1 : Terminator
  acc_x_drag_mDs2 : Outport  OutputWhenDisabled=reset  InitialOutput=0  VectorParamsAs1DForOutWhenUnconnected=off
  acc_y_drag_mDs2 : Outport  Port=2  OutputWhenDisabled=reset  InitialOutput=0  VectorParamsAs1DForOutWhenUnconnected=off
  acc_z_drag_mDs2 : Outport  Port=3  OutputWhenDisabled=reset  InitialOutput=0  VectorParamsAs1DForOutWhenUnconnected=off
  wires:
  alpha/1 -> Terminator/1
  beta/1 -> Terminator1/1
  Constant/1 -> acc_x_drag_mDs2/1
  Constant1/1 -> acc_y_drag_mDs2/1
  Constant2/1 -> acc_z_drag_mDs2/1

== system lib_FDM/FDM/FDM_Basic/Motion_Kinematics/Gravity ==
  note: derived from transformation matrix NED to Body
  note: for decoupling, set phi to zero??!!!
  phi : Inport
  theta : Inport  Port=2
  psi : Inport  Port=3
  Enable : EnablePort
  Constant1 : Constant  Value=FDM.Environment_Data.gravity_mDs2
  MATLAB Function : MATLAB Function  TreatAsAtomicUnit=on
  acc_x_grav_mDs : Outport  OutputWhenDisabled=reset  InitialOutput=0  VectorParamsAs1DForOutWhenUnconnected=off
  acc_y_grav_mDs : Outport  Port=2  OutputWhenDisabled=reset  InitialOutput=0  VectorParamsAs1DForOutWhenUnconnected=off
  acc_z_grav_mDs : Outport  Port=3  OutputWhenDisabled=reset  InitialOutput=0  VectorParamsAs1DForOutWhenUnconnected=off
  wires:
  Constant1/1 -> MATLAB Function/1(g)
  phi/1 -> MATLAB Function/2(phi)
  theta/1 -> MATLAB Function/3(theta)
  psi/1 -> MATLAB Function/4(psi)
  MATLAB Function/1(acc_x) -> acc_x_grav_mDs/1
  MATLAB Function/2(acc_y) -> acc_y_grav_mDs/1
  MATLAB Function/3(acc_z) -> acc_z_grav_mDs/1

== system lib_FDM/FDM/FDM_Basic/Motion_Kinematics/NED2PosWGS84Dot ==
  note: derived from Scriptum
  mue_rad : Inport
  h_m : Inport  Port=2
  x_dot_NED_mDs : Inport  Port=3
  y_dot_NED_mDs : Inport  Port=4
  z_dot_NED_mDs : Inport  Port=5
  MATLAB Function : MATLAB Function  TreatAsAtomicUnit=on
  lambda_dot_radDs : Outport  VectorParamsAs1DForOutWhenUnconnected=off
  mue_dot_radDs : Outport  Port=2  VectorParamsAs1DForOutWhenUnconnected=off
  h_dot_mDs : Outport  Port=3  VectorParamsAs1DForOutWhenUnconnected=off
  wires:
  h_m/1 -> MATLAB Function/5(h)
  mue_rad/1 -> MATLAB Function/4(mue)
  z_dot_NED_mDs/1 -> MATLAB Function/3(z_dot_NED)
  y_dot_NED_mDs/1 -> MATLAB Function/2(y_dot_NED)
  x_dot_NED_mDs/1 -> MATLAB Function/1(x_dot_NED)
  MATLAB Function/3(h_dot) -> h_dot_mDs/1
  MATLAB Function/2(mue_dot) -> mue_dot_radDs/1
  MATLAB Function/1(lambda_dot) -> lambda_dot_radDs/1

== system lib_FDM/FDM/FDM_Basic/Motion_Kinematics/Propulsion ==
  Motor_Ignition_flg : Inport
  Enable : EnablePort
  Add : Sum  Inputs=-+
  Clock : Clock
  Compare To Constant : simulink/Logic and Bit Operations/Compare To Constant  relop=<  const=FDM.Configuration_Data.Propulsion.burntime_s  OutDataTypeStr=boolean
  Logical Operator : Logic  Operator=NOT  AllPortsSameDT=off  OutDataTypeStr=boolean
  Logical Operator1 : Logic  Operator=OR  AllPortsSameDT=off  OutDataTypeStr=boolean
  Logical Operator2 : Logic  AllPortsSameDT=off  OutDataTypeStr=boolean
  Subsystem : Subsystem
  hold_time : Subsystem
  lock : Memory
  F_x_prop_N : Outport  VectorParamsAs1DForOutWhenUnconnected=off
  motor_state_perc_dot : Outport  Port=2  OutputWhenDisabled=reset  InitialOutput=0  VectorParamsAs1DForOutWhenUnconnected=off
  wires:
  Motor_Ignition_flg/1 -> Logical Operator1/1
  Logical Operator1/1 -> lock/1, Logical Operator/1, Logical Operator2/1
  lock/1 -> Logical Operator1/2
  Logical Operator/1 -> hold_time/Enable
  hold_time/1(exec_time_hold_s) -> Add/1
  Clock/1 -> Add/2
  Add/1 -> Compare To Constant/1, Subsystem/1(runtime)
  Subsystem/1(thrust) -> F_x_prop_N/1
  Subsystem/2(state_percentage_change) -> motor_state_perc_dot/1
  Compare To Constant/1 -> Logical Operator2/2
  Logical Operator2/1 -> Subsystem/Enable

== system lib_FDM/FDM/FDM_Basic/Motion_Kinematics/pqr2EulerDot ==
  ATT : Inport  OutDataTypeStr=Bus: ATT_Euler_Bus
  p : Inport  Port=2
  q : Inport  Port=3
  r : Inport  Port=4
  Add : Sum  Inputs=+++
  Add1 : Sum
  Add2 : Sum
  Bus Selector : BusSelector  OutputSignals=ATT_Phi_rad,ATT_Theta_rad
  Divide : Product  Inputs=*/
  Divide1 : Product  Inputs=*/
  Fcn1 : Fcn  Expr=-sin(u)
  Fcn{6,8,10..12} (5 alike) : Fcn  Expr=cos(u)
  Fcn4 : Fcn  Expr=sin(u)
  Fcn5 : Fcn  Expr=tan(u)
  Fcn7 : Fcn  Expr=tan(u)
  Fcn9 : Fcn  Expr=sin(u)
  Multiply{,1..7} (8 alike) : Product
  phi_dot : Outport  VectorParamsAs1DForOutWhenUnconnected=off
  theta_dot : Outport  Port=2  VectorParamsAs1DForOutWhenUnconnected=off
  psi_dot : Outport  Port=3  VectorParamsAs1DForOutWhenUnconnected=off
  wires:
  ATT/1 -> Bus Selector/1
  Add2/1 -> psi_dot/1
  Add1/1 -> theta_dot/1
  Add/1 -> phi_dot/1
  Fcn4/1 -> Multiply/1
  Fcn5/1 -> Multiply/2
  p/1 -> Add/1
  Bus Selector/1 -> Fcn1/1, Fcn8/1, Fcn6/1, Fcn4/1, Fcn11/1, Fcn9/1  "<ATT_Phi_rad>"
  Bus Selector/2 -> Fcn7/1, Fcn5/1, Fcn12/1, Fcn10/1  "<ATT_Theta_rad>"
  Fcn6/1 -> Multiply1/1
  Fcn7/1 -> Multiply1/2
  Fcn9/1 -> Divide/1
  Fcn10/1 -> Divide/2
  Fcn11/1 -> Divide1/1
  Fcn12/1 -> Divide1/2
  Multiply/1 -> Multiply2/2
  q/1 -> Multiply2/1, Multiply6/1, Multiply4/2
  Multiply2/1 -> Add/2
  Multiply1/1 -> Multiply3/2
  r/1 -> Multiply3/1, Multiply7/1, Multiply5/2
  Multiply3/1 -> Add/3
  Fcn8/1 -> Multiply4/1
  Fcn1/1 -> Multiply5/1
  Multiply4/1 -> Add1/1
  Multiply5/1 -> Add1/2
  Divide/1 -> Multiply6/2
  Divide1/1 -> Multiply7/2
  Multiply6/1 -> Add2/1
  Multiply7/1 -> Add2/2

== system lib_FDM/FDM/FDM_Basic/Motion_Kinematics/uvw2PosNEDDot ==
  note: for decoupling, set phi to zero??!!!
  note: derived from Rotation Matrix Body Frame to NED Frame
  u : Inport
  v : Inport  Port=2
  w : Inport  Port=3
  ATT : Inport  Port=4  OutDataTypeStr=Bus: ATT_Euler_Bus
  Bus Selector : BusSelector  OutputSignals=ATT_Phi_rad,ATT_Theta_rad,ATT_Psi_rad
  MATLAB Function : MATLAB Function  TreatAsAtomicUnit=on
  MATLAB Function1 : MATLAB Function  TreatAsAtomicUnit=on
  MATLAB Function2 : MATLAB Function  TreatAsAtomicUnit=on
  x_dot_mDs : Outport  VectorParamsAs1DForOutWhenUnconnected=off
  y_dot_mDs : Outport  Port=2  VectorParamsAs1DForOutWhenUnconnected=off
  z_dot_mDs : Outport  Port=3  VectorParamsAs1DForOutWhenUnconnected=off
  wires:
  ATT/1 -> Bus Selector/1
  u/1 -> MATLAB Function2/1(u), MATLAB Function1/1(u), MATLAB Function/1(u)
  v/1 -> MATLAB Function2/2(v), MATLAB Function1/2(v), MATLAB Function/2(v)
  w/1 -> MATLAB Function2/3(w), MATLAB Function1/3(w), MATLAB Function/3(w)
  Bus Selector/1 -> MATLAB Function2/4(phi), MATLAB Function1/4(phi), MATLAB Function/4(phi)  "<ATT_Phi_rad>"
  Bus Selector/2 -> MATLAB Function2/5(theta), MATLAB Function1/5(theta), MATLAB Function/5(theta)  "<ATT_Theta_rad>"
  Bus Selector/3 -> MATLAB Function1/6(psi), MATLAB Function/6(psi)  "<ATT_Psi_rad>"
  MATLAB Function/1(N_dot) -> x_dot_mDs/1
  MATLAB Function1/1(E_dot) -> y_dot_mDs/1
  MATLAB Function2/1(D_dot) -> z_dot_mDs/1

== system lib_FDM/FDM/FDM_Basic/State_Integration/ATT_Integration ==
  Simulation_Control : Inport  OutDataTypeStr=Bus: Simulation_Ctrl_Bus
  Initial_States : Inport  Port=2  OutDataTypeStr=Bus: States_Bus
  phi_dot_radDs : Inport  Port=3
  theta_dot_radDs : Inport  Port=4
  psi_dot_radDs : Inport  Port=5
  Bus Selector : BusSelector  OutputSignals=run,reset
  Bus Selector1 : BusSelector  OutputSignals=Rigid_Body_States.Attitude_States.ATT_Euler.ATT_Phi_rad
  Bus Selector2 : BusSelector  OutputSignals=Rigid_Body_States.Attitude_States.ATT_Euler.ATT_Theta_rad
  Bus Selector3 : BusSelector  OutputSignals=Rigid_Body_States.Attitude_States.ATT_Euler.ATT_Psi_rad
  Data Type Conversion : DataTypeConversion  OutDataTypeStr=double
  Integrator : Integrator  ExternalReset=rising  InitialConditionSource=external
  Integrator1 : Integrator  ExternalReset=rising  InitialConditionSource=external
  Integrator2 : Integrator  ExternalReset=rising  InitialConditionSource=external
  Product : Product
  Product1 : Product
  Product2 : Product
  phi_rad : Outport  VectorParamsAs1DForOutWhenUnconnected=off
  theta_rad : Outport  Port=2  VectorParamsAs1DForOutWhenUnconnected=off
  psi_rad : Outport  Port=3  VectorParamsAs1DForOutWhenUnconnected=off
  wires:
  Simulation_Control/1 -> Bus Selector/1
  Bus Selector/1 -> Data Type Conversion/1  "<run>"
  Data Type Conversion/1 -> Product/2, Product1/2, Product2/2
  Product/1 -> Integrator/1
  psi_dot_radDs/1 -> Product2/1
  theta_dot_radDs/1 -> Product1/1
  phi_dot_radDs/1 -> Product/1
  Bus Selector/2 -> Integrator2/2, Integrator1/2, Integrator/2  "<reset>"
  Bus Selector1/1 -> Integrator/3  "<ATT_Phi_rad>"
  Product1/1 -> Integrator1/1
  Initial_States/1 -> Bus Selector3/1, Bus Selector2/1, Bus Selector1/1
  Product2/1 -> Integrator2/1
  Integrator/1 -> phi_rad/1
  Integrator1/1 -> theta_rad/1
  Integrator2/1 -> psi_rad/1
  Bus Selector3/1 -> Integrator2/3  "<ATT_Psi_rad>"
  Bus Selector2/1 -> Integrator1/3  "<ATT_Theta_rad>"

== system lib_FDM/FDM/FDM_Basic/State_Integration/Mass_Balance ==
  note: linear interpolation between initial and burnout values of inertia and mass
  motor_state_perc : Inport
  Add{,1..3} (4 alike) : Sum
  Constant : Constant  Value=FDM.Configuration_Data.mass_preburn_kg-FDM.Configuration_Data.mass_kg
  Constant1 : Constant  Value=FDM.Configuration_Data.mass_kg
  Constant2 : Constant  Value=FDM.Configuration_Data.I_x_kgDm2
  Constant3 : Constant  Value=FDM.Configuration_Data.I_x_preburn_kgDm2-FDM.Configuration_Data.I_x_kgDm2
  Constant4 : Constant  Value=FDM.Configuration_Data.I_y_kgDm2
  Constant5 : Constant  Value=FDM.Configuration_Data.I_y_preburn_kgDm2-FDM.Configuration_Data.I_y_kgDm2
  Constant6 : Constant  Value=FDM.Configuration_Data.I_z_kgDm2
  Constant7 : Constant  Value=FDM.Configuration_Data.I_z_preburn_kgDm2-FDM.Configuration_Data.I_z_kgDm2
  Multiply{,1..3} (4 alike) : Product
  mass_kg : Outport  VectorParamsAs1DForOutWhenUnconnected=off
  I_x_kgm2 : Outport  Port=2  VectorParamsAs1DForOutWhenUnconnected=off
  I_y_kgm2 : Outport  Port=3  VectorParamsAs1DForOutWhenUnconnected=off
  I_z_kgm2 : Outport  Port=4  VectorParamsAs1DForOutWhenUnconnected=off
  wires:
  Constant1/1 -> Add/1
  Constant/1 -> Multiply/2
  Multiply/1 -> Add/2
  motor_state_perc/1 -> Multiply1/1, Multiply2/1, Multiply3/1, Multiply/1
  Add/1 -> mass_kg/1
  Constant3/1 -> Multiply1/2
  Multiply1/1 -> Add1/2
  Constant2/1 -> Add1/1
  Constant5/1 -> Multiply2/2
  Constant4/1 -> Add2/1
  Multiply2/1 -> Add2/2
  Constant6/1 -> Add3/1
  Constant7/1 -> Multiply3/2
  Multiply3/1 -> Add3/2
  Add1/1 -> I_x_kgm2/1
  Add2/1 -> I_y_kgm2/1
  Add3/1 -> I_z_kgm2/1

== system lib_FDM/FDM/FDM_Basic/State_Integration/Motor_State_Integration ==
  Simulation_Control : Inport  OutDataTypeStr=Bus: Simulation_Ctrl_Bus
  Initial_States : Inport  Port=2  OutDataTypeStr=Bus: States_Bus
  motor_state_dot_percDs : Inport  Port=3
  Bus Selector2 : BusSelector  OutputSignals=Airframe_States.motor_state_perc
  Bus Selector3 : BusSelector  OutputSignals=run,reset
  Data Type Conversion : DataTypeConversion  OutDataTypeStr=double
  Integrator : Integrator  ExternalReset=rising  InitialConditionSource=external
  Multiply : Product
  motor_state_perc : Outport  VectorParamsAs1DForOutWhenUnconnected=off
  wires:
  Bus Selector2/1 -> Integrator/3  "<motor_state_perc>"
  Bus Selector3/2 -> Integrator/2  "<reset>"
  Bus Selector3/1 -> Data Type Conversion/1  "<run>"
  motor_state_dot_percDs/1 -> Multiply/1
  Integrator/1 -> motor_state_perc/1
  Multiply/1 -> Integrator/1
  Simulation_Control/1 -> Bus Selector3/1
  Initial_States/1 -> Bus Selector2/1
  Data Type Conversion/1 -> Multiply/2

== system lib_FDM/FDM/FDM_Basic/State_Integration/POS_NED_Integrator ==
  Simulation_Control : Inport  OutDataTypeStr=Bus: Simulation_Ctrl_Bus
  Initial_States : Inport  Port=2  OutDataTypeStr=Bus: States_Bus
  x_dot_mDs : Inport  Port=3
  y_dot_mDs : Inport  Port=4
  z_dot_mDs : Inport  Port=5
  Bus Selector : BusSelector  OutputSignals=run,reset
  Bus Selector1 : BusSelector  OutputSignals=Rigid_Body_States.Position_States.POS_NED.POS_x_NED_m
  Bus Selector2 : BusSelector  OutputSignals=Rigid_Body_States.Position_States.POS_NED.POS_y_NED_m
  Bus Selector3 : BusSelector  OutputSignals=Rigid_Body_States.Position_States.POS_NED.POS_z_NED_m
  Data Type Conversion : DataTypeConversion  OutDataTypeStr=double
  Integrator : Integrator  ExternalReset=rising  InitialConditionSource=external
  Integrator1 : Integrator  ExternalReset=rising  InitialConditionSource=external
  Integrator2 : Integrator  ExternalReset=rising  InitialConditionSource=external
  Product : Product
  Product1 : Product
  Product2 : Product
  x_m : Outport  VectorParamsAs1DForOutWhenUnconnected=off
  y_m : Outport  Port=2  VectorParamsAs1DForOutWhenUnconnected=off
  z_m : Outport  Port=3  VectorParamsAs1DForOutWhenUnconnected=off
  wires:
  Simulation_Control/1 -> Bus Selector/1
  Bus Selector/1 -> Data Type Conversion/1  "<run>"
  Data Type Conversion/1 -> Product/2, Product1/2, Product2/2
  Product/1 -> Integrator/1
  z_dot_mDs/1 -> Product2/1
  y_dot_mDs/1 -> Product1/1
  x_dot_mDs/1 -> Product/1
  Bus Selector/2 -> Integrator2/2, Integrator1/2, Integrator/2  "<reset>"
  Bus Selector1/1 -> Integrator/3  "<POS_x_NED_m>"
  Product1/1 -> Integrator1/1
  Initial_States/1 -> Bus Selector3/1, Bus Selector2/1, Bus Selector1/1
  Product2/1 -> Integrator2/1
  Integrator/1 -> x_m/1
  Integrator1/1 -> y_m/1
  Integrator2/1 -> z_m/1
  Bus Selector3/1 -> Integrator2/3  "<POS_z_NED_m>"
  Bus Selector2/1 -> Integrator1/3  "<POS_y_NED_m>"

== system lib_FDM/FDM/FDM_Basic/State_Integration/POS_WGS84_Integrator ==
  Simulation_Control : Inport  OutDataTypeStr=Bus: Simulation_Ctrl_Bus
  Initial_States : Inport  Port=2  OutDataTypeStr=Bus: States_Bus
  lambda_dot_radDs : Inport  Port=3
  mue_dot_radDs : Inport  Port=4
  h_dot_mDs : Inport  Port=5
  Bus Selector : BusSelector  OutputSignals=run,reset
  Bus Selector1 : BusSelector  OutputSignals=Rigid_Body_States.Position_States.POS_WGS84.POS_lambda_WGS84_rad
  Bus Selector2 : BusSelector  OutputSignals=Rigid_Body_States.Position_States.POS_WGS84.POS_mue_WGS84_rad
  Bus Selector3 : BusSelector  OutputSignals=Rigid_Body_States.Position_States.POS_WGS84.POS_h_WGS84_m
  Data Type Conversion : DataTypeConversion  OutDataTypeStr=double
  Integrator : Integrator  ExternalReset=rising  InitialConditionSource=external
  Integrator1 : Integrator  ExternalReset=rising  InitialConditionSource=external
  Integrator2 : Integrator  ExternalReset=rising  InitialConditionSource=external
  Product : Product
  Product1 : Product
  Product2 : Product
  lambda_rad : Outport  VectorParamsAs1DForOutWhenUnconnected=off
  mue_rad : Outport  Port=2  VectorParamsAs1DForOutWhenUnconnected=off
  h_m : Outport  Port=3  VectorParamsAs1DForOutWhenUnconnected=off
  wires:
  Simulation_Control/1 -> Bus Selector/1
  Bus Selector/1 -> Data Type Conversion/1  "<run>"
  Data Type Conversion/1 -> Product/2, Product1/2, Product2/2
  Product/1 -> Integrator/1
  h_dot_mDs/1 -> Product2/1
  mue_dot_radDs/1 -> Product1/1
  lambda_dot_radDs/1 -> Product/1
  Bus Selector/2 -> Integrator2/2, Integrator1/2, Integrator/2  "<reset>"
  Bus Selector1/1 -> Integrator/3  "<POS_lambda_WGS84_rad>"
  Product1/1 -> Integrator1/1
  Initial_States/1 -> Bus Selector3/1, Bus Selector2/1, Bus Selector1/1
  Product2/1 -> Integrator2/1
  Integrator/1 -> lambda_rad/1
  Integrator1/1 -> mue_rad/1
  Integrator2/1 -> h_m/1
  Bus Selector3/1 -> Integrator2/3  "<POS_h_WGS84_m>"
  Bus Selector2/1 -> Integrator1/3  "<POS_mue_WGS84_rad>"
